simulink model "MED2018_VehicleModel_Example_tested"  (R2017b)
settings: Solver=FixedStepDiscrete  StartTime=0.0  StopTime=30  FixedStep=0.01  RelTol=1e-3
libraries: simulink x3
settings Model: SimulationMode=accelerator  Creator=ashwin.ramanujam  LastModifiedBy=Lenovo g505s

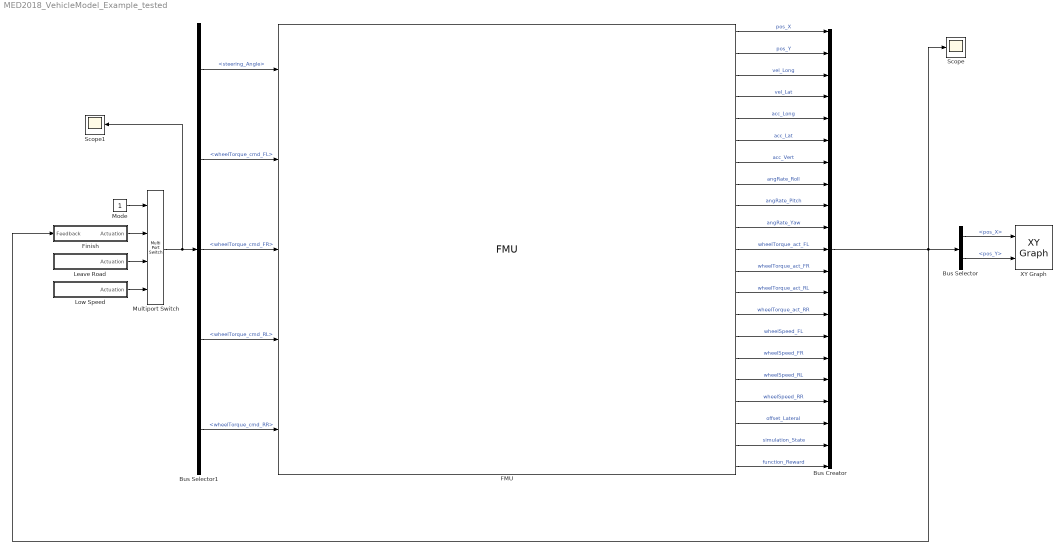
== system MED2018_VehicleModel_Example_tested ==
  Bus Creator : BusCreator  Inputs=21
  Bus Selector : BusSelector  OutputSignals=pos_X,pos_Y
  Bus Selector1 : BusSelector  OutputSignals=steering_Angle,wheelTorque_cmd_FL,wheelTorque_cmd_FR,wheelTorque_cmd_RL,wheelTorque_cmd_RR
  FMU : FMU  FMUName=MED2018_VehicleModel.fmu  FMUDebugLogging=on  FMUMode=CoSimulation  FMUSampleTime=-1  mask(MED2018.VehicleModel [Co-Simulation, v2.0]){}
      mask Display:
      | if (exist([Simulink.fileGenControl('get','CacheFolder') '\slprj\_fmu\61fc1e840d73583fbd52d6718d3f74dd\MED2018_VehicleModel\model.png'],'file'))
      |     image([Simulink.fileGenControl('get','CacheFolder') '\slprj\_fmu\61fc1e840d73583fbd52d6718d3f74dd\MED2018_VehicleModel\model.png']);
      |     text(0.03, 0.97, 'MED2018.VehicleModel', 'horizontalAlignment', 'left', 'verticalAlignment', 'top');
      | else
      |     disp('MED2018.VehicleModel');
      | end
      | port_label('output',1,'pos_X');
      | port_label('output',2,'pos_Y');
      | port_label('output',3,'vel_Long');
      | port_label('output',4,'vel_Lat');
      | port_label('output',5,'acc_Long');
      | port_label('output',6,'acc_Lat');
      | port_label('output',7,'acc_Vert');
      | port_label('output',8,'angRate_Roll');
      | port_label('output',9,'angRate_Pitch');
      | port_label('output',10,'angRate_Yaw');
      | port_label('output',11,'wheellTorque_act_FL');
      | port_label('output',12,'wheelTorque_act_FR');
      | port_label('output',13,'wheelTorque_act_RL');
      | port_label('output',14,'wheelTorque_act_RR');
      | port_label('output',15,'wheelSpeed_FL');
      | port_label('output',16,'wheelSpeed_FR');
      | port_label('output',17,'wheelSpeed_RL');
      | port_label('output',18,'wheelSpeed_RR');
      | port_label('output',19,'offset_Lateral');
      | port_label('output',20,'simulation_State');
      | port_label('output',21,'function_Reward');
      | port_label('input',1,'steering_Angle');
      | port_label('input',2,'wheelTorque_cmd_FL');
      | port_label('input',3,'wheelTorque_cmd_FR');
      | port_label('input',4,'wheelTorque_cmd_RL');
      | port_label('input',5,'wheelTorque_cmd_RR');
  Finish : Subsystem
  Leave Road : Subsystem
  Low Speed : Subsystem
  Mode : Constant
  Multiport Switch : MultiPortSwitch
  Scope : Scope
  Scope1 : Scope
  XY Graph : simulink/Sinks/XY Graph  xmin=-1  xmax=110  ymin=-1  ymax=180  st=-1
  wires:
  Multiport Switch/1 -> Scope1/1, Bus Selector1/1
  Finish/1(Actuation) -> Multiport Switch/2
  Mode/1 -> Multiport Switch/1
  Bus Selector1/1 -> FMU/1  "<steering_Angle>"
  Bus Selector1/2 -> FMU/2  "<wheelTorque_cmd_FL>"
  Bus Selector1/3 -> FMU/3  "<wheelTorque_cmd_FR>"
  Bus Selector1/4 -> FMU/4  "<wheelTorque_cmd_RL>"
  Bus Selector1/5 -> FMU/5  "<wheelTorque_cmd_RR>"
  FMU/1 -> Bus Creator/1  "pos_X"
  FMU/2 -> Bus Creator/2  "pos_Y"
  FMU/3 -> Bus Creator/3  "vel_Long"
  FMU/4 -> Bus Creator/4  "vel_Lat"
  FMU/5 -> Bus Creator/5  "acc_Long"
  FMU/6 -> Bus Creator/6  "acc_Lat"
  FMU/7 -> Bus Creator/7  "acc_Vert"
  FMU/8 -> Bus Creator/8  "angRate_Roll"
  FMU/9 -> Bus Creator/9  "angRate_Pitch"
  FMU/10 -> Bus Creator/10  "angRate_Yaw"
  FMU/11 -> Bus Creator/11  "wheelTorque_act_FL"
  FMU/12 -> Bus Creator/12  "wheelTorque_act_FR"
  FMU/13 -> Bus Creator/13  "wheelTorque_act_RL"
  FMU/14 -> Bus Creator/14  "wheelTorque_act_RR"
  FMU/15 -> Bus Creator/15  "wheelSpeed_FL"
  FMU/16 -> Bus Creator/16  "wheelSpeed_FR"
  FMU/17 -> Bus Creator/17  "wheelSpeed_RL"
  FMU/18 -> Bus Creator/18  "wheelSpeed_RR"
  FMU/19 -> Bus Creator/19  "offset_Lateral"
  FMU/20 -> Bus Creator/20  "simulation_State"
  FMU/21 -> Bus Creator/21  "function_Reward"
  Bus Selector/1 -> XY Graph/1  "<pos_X>"
  Bus Selector/2 -> XY Graph/2  "<pos_Y>"
  Bus Creator/1 -> Scope/1, Finish/1(Feedback), Bus Selector/1
  Leave Road/1(Actuation) -> Multiport Switch/3
  Low Speed/1(Actuation) -> Multiport Switch/4

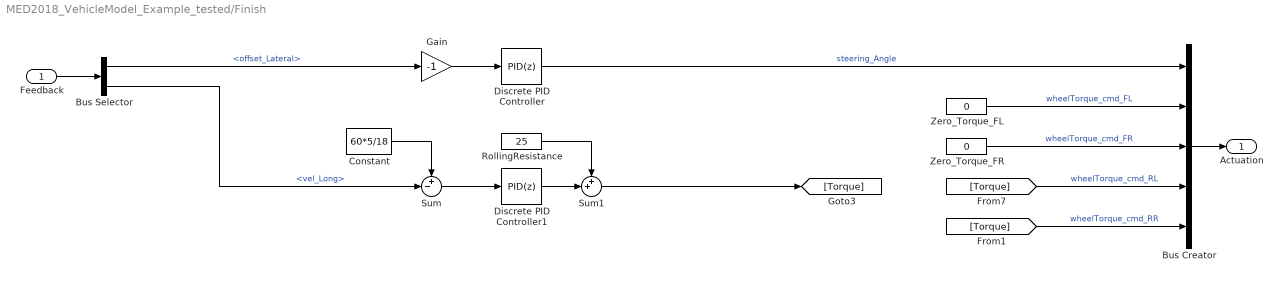
== system MED2018_VehicleModel_Example_tested/Finish ==
  Feedback : Inport
  Bus Creator : BusCreator  Inputs=5
  Bus Selector : BusSelector  OutputSignals=offset_Lateral,vel_Long
  Constant : Constant  Value=60*5/18
  Discrete PID Controller : simulink/Continuous/PID Controller  Controller=PID  TimeDomain=Discrete-time  SampleTime=-1  IntegratorMethod=Forward Euler  FilterMethod=Forward Euler  Form=Parallel  UseFilter=off  ControllerParametersSource=internal  P=1  I=0  D=1  N=100  InitialConditionSource=internal  InitialConditionForIntegrator=0  InitialConditionForFilter=0  ExternalReset=none  LimitOutput=off  UpperSaturationLimit=inf  LowerSaturationLimit=-inf  LinearizeAsGain=off  AntiWindupMode=none  Kb=1  TrackingMode=off  Kt=1  PParamMin=[]  PParamMax=[]  IParamMin=[]  IParamMax=[]  DParamMin=[]  DParamMax=[]  NParamMin=[]  NParamMax=[]  KbParamMin=[]  KbParamMax=[]  KtParamMin=[]  KtParamMax=[]  POutMin=[]  POutMax=[]  IOutMin=[]  IOutMax=[]  DOutMin=[]  DOutMax=[]  NOutMin=[]  NOutMax=[]  KbOutMin=[]  KbOutMax=[]  KtOutMin=[]  KtOutMax=[]  IntegratorOutMin=[]  IntegratorOutMax=[]  FilterOutMin=[]  FilterOutMax=[]  SumOutMin=[]  SumOutMax=[]  SumI1OutMin=[]  SumI1OutMax=[]  SumI2OutMin=[]  SumI2OutMax=[]  SumI3OutMin=[]  SumI3OutMax=[]  SumDOutMin=[]  SumDOutMax=[]  SaturationOutMin=[]  SaturationOutMax=[]  IntegratorContinuousStateAttributes=''  IntegratorStateMustResolveToSignalObject=off  IntegratorRTWStateStorageClass=Auto  FilterContinuousStateAttributes=''  FilterStateMustResolveToSignalObject=off  FilterRTWStateStorageClass=Auto  DifferentiatorICPrevScaledInput=0  DifferentiatorOutMin=[]  DifferentiatorOutMax=[]  InitialConditionSetting=State (most efficient)  FilterDiffOutCoefMin=[]  FilterDiffOutCoefMax=[]  SumDenOutMin=[]  SumDenOutMax=[]  SumNumOutMin=[]  SumNumOutMax=[]  ReciprocalOutMin=[]  ReciprocalOutMax=[]  DivideOutMin=[]  DivideOutMax=[]  TunerSelectOption=Transfer Function Based (PID Tuner App)
  Discrete PID Controller1 : simulink/Continuous/PID Controller  Controller=PID  TimeDomain=Discrete-time  SampleTime=-1  IntegratorMethod=Forward Euler  FilterMethod=Forward Euler  Form=Parallel  UseFilter=on  ControllerParametersSource=internal  P=100  I=0  D=0.1  N=100  InitialConditionSource=internal  InitialConditionForIntegrator=0  InitialConditionForFilter=0  ExternalReset=none  LimitOutput=off  UpperSaturationLimit=inf  LowerSaturationLimit=-inf  LinearizeAsGain=off  AntiWindupMode=none  Kb=1  TrackingMode=off  Kt=1  PParamMin=[]  PParamMax=[]  IParamMin=[]  IParamMax=[]  DParamMin=[]  DParamMax=[]  NParamMin=[]  NParamMax=[]  KbParamMin=[]  KbParamMax=[]  KtParamMin=[]  KtParamMax=[]  POutMin=[]  POutMax=[]  IOutMin=[]  IOutMax=[]  DOutMin=[]  DOutMax=[]  NOutMin=[]  NOutMax=[]  KbOutMin=[]  KbOutMax=[]  KtOutMin=[]  KtOutMax=[]  IntegratorOutMin=[]  IntegratorOutMax=[]  FilterOutMin=[]  FilterOutMax=[]  SumOutMin=[]  SumOutMax=[]  SumI1OutMin=[]  SumI1OutMax=[]  SumI2OutMin=[]  SumI2OutMax=[]  SumI3OutMin=[]  SumI3OutMax=[]  SumDOutMin=[]  SumDOutMax=[]  SaturationOutMin=[]  SaturationOutMax=[]  IntegratorContinuousStateAttributes=''  IntegratorStateMustResolveToSignalObject=off  IntegratorRTWStateStorageClass=Auto  FilterContinuousStateAttributes=''  FilterStateMustResolveToSignalObject=off  FilterRTWStateStorageClass=Auto  DifferentiatorICPrevScaledInput=0  DifferentiatorOutMin=[]  DifferentiatorOutMax=[]  InitialConditionSetting=State (most efficient)  FilterDiffOutCoefMin=[]  FilterDiffOutCoefMax=[]  SumDenOutMin=[]  SumDenOutMax=[]  SumNumOutMin=[]  SumNumOutMax=[]  ReciprocalOutMin=[]  ReciprocalOutMax=[]  DivideOutMin=[]  DivideOutMax=[]  TunerSelectOption=Transfer Function Based (PID Tuner App)
  Gain : Gain  Gain=-1
  RollingResistance : Constant  Value=25
  Sum : Sum  Inputs=+-|
  Sum1 : Sum  Inputs=++|
  Zero_Torque_FL : Constant  Value=0
  Zero_Torque_FR : Constant  Value=0
  Actuation : Outport
  wires:
  Bus Creator/1 -> Actuation/1
  Gain/1 -> Discrete PID Controller/1
  Sum/1 -> Discrete PID Controller1/1
  Feedback/1 -> Bus Selector/1
  Sum1/1 -> [Torque]
  Bus Selector/2 -> Sum/2  "<vel_Long>"
  Constant/1 -> Sum/1
  Bus Selector/1 -> Gain/1  "<offset_Lateral>"
  Discrete PID Controller/1 -> Bus Creator/1  "steering_Angle"
  Discrete PID Controller1/1 -> Sum1/2
  RollingResistance/1 -> Sum1/1
  Zero_Torque_FL/1 -> Bus Creator/2  "wheelTorque_cmd_FL"
  [Torque] -> Bus Creator/4  "wheelTorque_cmd_RL"
  Zero_Torque_FR/1 -> Bus Creator/3  "wheelTorque_cmd_FR"
  [Torque] -> Bus Creator/5  "wheelTorque_cmd_RR"

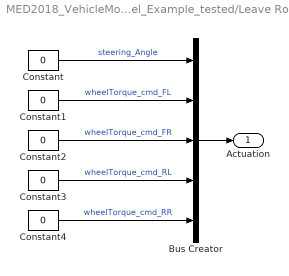
== system MED2018_VehicleModel_Example_tested/Leave Road ==
  Bus Creator : BusCreator  Inputs=5
  Constant{,1..4} (5 alike) : Constant  Value=0
  Actuation : Outport
  wires:
  Constant4/1 -> Bus Creator/5  "wheelTorque_cmd_RR"
  Constant1/1 -> Bus Creator/2  "wheelTorque_cmd_FL"
  Constant3/1 -> Bus Creator/4  "wheelTorque_cmd_RL"
  Constant/1 -> Bus Creator/1  "steering_Angle"
  Constant2/1 -> Bus Creator/3  "wheelTorque_cmd_FR"
  Bus Creator/1 -> Actuation/1

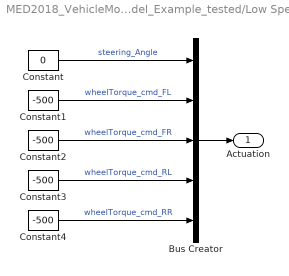
== system MED2018_VehicleModel_Example_tested/Low Speed ==
  Bus Creator : BusCreator  Inputs=5
  Constant : Constant  Value=0
  Constant{1..4} (4 alike) : Constant  Value=-500
  Actuation : Outport
  wires:
  Bus Creator/1 -> Actuation/1
  Constant3/1 -> Bus Creator/4  "wheelTorque_cmd_RL"
  Constant1/1 -> Bus Creator/2  "wheelTorque_cmd_FL"
  Constant/1 -> Bus Creator/1  "steering_Angle"
  Constant4/1 -> Bus Creator/5  "wheelTorque_cmd_RR"
  Constant2/1 -> Bus Creator/3  "wheelTorque_cmd_FR"
